simulink model "CompFilter_testHarness"  (R2012b)
settings: Solver=FixedStepDiscrete  StartTime=0.0  StopTime=50  RelTol=1e-3
InitFcn:
  | p = fileparts(which(bdroot));
  | load(fullfile(p,'CompFilter_testData'))
values from neighbouring files (symbols this model uses):
  F_LUT =     [CompFilter_testData.mat]    (also in filterResponseData.m = [])
undefined symbols (not defined in the file or in its folder): sigbuilder_block
libraries: simulink x13, ResultLoggerLib x4
settings Model: RequirementInfo={'other' '..\..\..\..\requirements\ebd_srs.doc' '@Simulink_requirement_item_4' 'true' 'REQ001- Filter input signal via polyphase digital filter bank' 'Requirement' } %GIDa_bfa4a348_cd9f_4101_a776_3ea215f34dae  SldvGeneratedHarnessModel=TestUnitModel=CompFeatures|  RecordCoverage=on  CovMetricSettings=dcmtroie  CovHTMLOptions=-sRT=1 -aTS=1 -bRG=1 -bTC=0 -hTR=0 -nFC=0 -scm=1 -bcm=1 -xEv=0  CovExternalEMLEnable=on  Creator=aanantha  LastModifiedBy=klindqvi
settings DataIOCC: SaveFormat=Structure  SignalLoggingSaveFormat=ModelDataLogs  SaveOutput=off  SaveTime=off  SignalLoggingName=logsOut
settings OptimizationCC: InlineParams=on  OptimizeModelRefInitCode=on  LifeSpan=1
settings DebuggingCC: ReadBeforeWriteMsg=DisableAll  WriteAfterWriteMsg=DisableAll  WriteAfterReadMsg=DisableAll  CheckSSInitialOutputMsg=off  SolverPrmCheckMsg=none  InheritedTsInSrcMsg=none  ParameterPrecisionLossMsg=none  FcnCallInpInsideContextMsg=EnableAllAsWarning  ModelReferenceSymbolNameMessage=none
settings HardwareCC: ProdLargestAtomicInteger=Long  ProdLargestAtomicFloat=Double  ProdEndianess=LittleEndian  ProdHWDeviceType=ARM Compatible->ARM Cortex
settings ModelReferenceCC: UpdateModelReferenceTargets=Force  CheckModelReferenceTargetMessage=none
settings RTWCC: SystemTargetFile=ert.tlc  TemplateMakefile=ert_default_tmf  Description=Embedded Coder  GenerateReport=on  ProcessScript=ert_make_rtw_hook  IncludeHyperlinkInReport=on  LaunchReport=on  GenerateTraceInfo=on  GenerateTraceReportSl=on  GenerateTraceReportSf=on  GenerateTraceReportEml=on  GenerateCodeMetricsReport=on
settings CodeAppCC: IgnoreCustomStorageClasses=off
settings ERTTargetCC: CodeReplacementLibrary=GCC ARM Cortex-A8  MultiwordLength=2048  GenerateSampleERTMain=on  ERTCustomFileTemplate=example_file_process.tlc  ConvertIfToSwitch=off  SuppressUnreachableDefaultCases=off

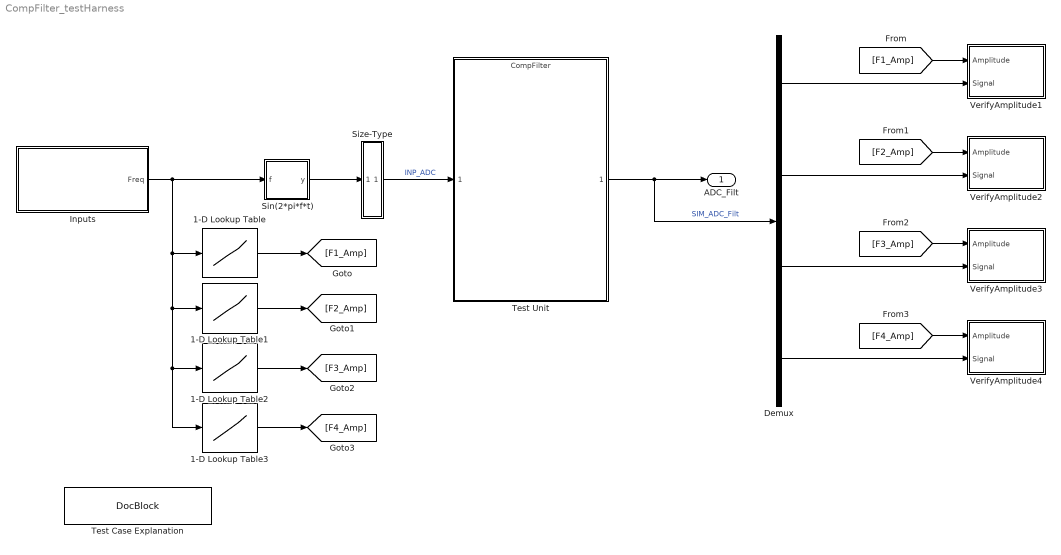
== system CompFilter_testHarness ==
  1-D Lookup Table : Lookup_n-D  NumberOfTableDimensions=1  BreakpointsForDimension1=F_LUT(1).bp  Table=F_LUT(1).table  InterpMethod=Cubic spline  RndMeth=Simplest  InputSameDT=on
  1-D Lookup Table1 : Lookup_n-D  NumberOfTableDimensions=1  BreakpointsForDimension1=F_LUT(2).bp  Table=F_LUT(2).table  InterpMethod=Cubic spline  RndMeth=Simplest  InputSameDT=on
  1-D Lookup Table2 : Lookup_n-D  NumberOfTableDimensions=1  BreakpointsForDimension1=F_LUT(3).bp  Table=F_LUT(3).table  InterpMethod=Cubic spline  RndMeth=Simplest  InputSameDT=on
  1-D Lookup Table3 : Lookup_n-D  NumberOfTableDimensions=1  BreakpointsForDimension1=F_LUT(4).bp  Table=F_LUT(4).table  InterpMethod=Cubic spline  RndMeth=Simplest  InputSameDT=on
  Demux : Demux
  Inputs : Subsystem  Tag=STV Subsys  RequirementInfo={'other' '..\..\..\..\requirements\ebd_srs.doc' '@REQ001- Filter input signal via polyphase digital filter bank' 'true' 'REQ001- Filter input signal via polyphase digital filter bank' '' ; 'other' '..\..\..\..\requirements\ebd_srs.doc' '@REQ001- Filter input signal via polyphase digital filter bank' 'true' 'REQ001- Filter input signal via polyphase digital filter bank' '' ; 'other' '..\..\..\..\requirements\ebd_srs.doc' '@REQ001- Filter input signal via polyphase digital filter bank' 'true' 'REQ001- Filter input signal via polyphase digital filter bank' '' ; 'other' '..\..\..\..\requirements\ebd_srs.doc' '@REQ001- Filter input signal via polyphase digital filter bank' 'true' 'REQ001- Filter input signal via polyphase digital filter bank' '' ; 'other' '..\..\..\..\requirements\ebd_srs.doc' '@REQ001- Filter input signal via polyphase digital filter bank' 'true' 'REQ001- Filter input signal via polyphase digital filter bank' '' ; 'other' '..\..\..\..\requirements\ebd_srs.doc' '@REQ001- Filter input signal via polyphase digital filter bank' 'true' 'REQ001- Filter input signal via polyphase digital filter bank' '' ; 'other' '..\..\..\..\requirements\ebd_srs.doc' '@REQ001- Filter input signal via polyphase digital filter bank' 'true' 'REQ001- Filter input signal via polyphase digital filter bank' '' } %GIDa_3ed100c0_3913_49f9_991c_94aec2cdfde7  LoadFcn=sigbuilder_block('load');  StartFcn=sigbuilder_block('start');  StopFcn=sigbuilder_block('stop');  ClipboardFcn=sigbuilder_block('clipboard');  mask(Sigbuilder block){}
      mask init:
      | if ~strcmp(get_param(bdroot(gcb),'SimulationStatus'),'stopped'),tuvar = sigbuilder_block('maskInit'); end
      settings: CopyFcn=sigbuilder_block('copy');  DeleteFcn=sigbuilder_block('delete');  ModelCloseFcn=sigbuilder_block('modelClose');  PreSaveFcn=sigbuilder_block('preSave');  PauseFcn=sigbuilder_block('pause');  ContinueFcn=sigbuilder_block('continue');  NameChangeFcn=sigbuilder_block('namechange');  OpenFcn=sigbuilder_block('open',[726.75 262.5 605.25 528 ]);  CloseFcn=sigbuilder_block('close');
      mask Display: plot(0, 0, 100, 100,[2, 2, 32, 32, 2], [68, 8, 8, 68, 68],[32, 2], [38, 38], [32, 19, 2],[53, 60, 44], [32, 17, 17, 2],[16, 16, 31, 31]);txt = getActiveGroup(gcbh);text(2, 100, txt,'verticalAlignment', 'top');
  Sin(2*pi*f*t) : Subsystem
  Size-Type : Subsystem
  Test Case Explanation : simulink/Model-Wide Utilities/DocBlock  DocumentType=Text
      content=|
      | Test case with default values because no SLDVDATA supplied
  Test Unit : ModelReference  ModelNameDialog=CompFilter  SimulationMode=Normal  ModelReferenceVersion=1.283  CopyOfModelName=CompFilter  DefaultDataLogging=on
  VerifyAmplitude1 : Subsystem
  VerifyAmplitude2 : Subsystem
  VerifyAmplitude3 : Subsystem
  VerifyAmplitude4 : Subsystem
  ADC_Filt : Outport  OutDataTypeStr=single  PortDimensions=4  SampleTime=[0.08900000000000001,0]
  wires:
  Size-Type/1(Out1) -> Test Unit/1  "INP_ADC"
  Test Unit/1 -> Demux/1, ADC_Filt/1  "SIM_ADC_Filt"
  [F1_Amp] -> VerifyAmplitude1/1(Amplitude)
  [F2_Amp] -> VerifyAmplitude2/1(Amplitude)
  Inputs/1(Freq) -> 1-D Lookup Table3/1, 1-D Lookup Table2/1, 1-D Lookup Table1/1, 1-D Lookup Table/1, Sin(2*pi*f*t)/1(f)
  Sin(2*pi*f*t)/1(y) -> Size-Type/1(In1)
  Demux/1 -> VerifyAmplitude1/2(Signal)
  Demux/2 -> VerifyAmplitude2/2(Signal)
  1-D Lookup Table/1 -> [F1_Amp]
  1-D Lookup Table1/1 -> [F2_Amp]
  1-D Lookup Table2/1 -> [F3_Amp]
  1-D Lookup Table3/1 -> [F4_Amp]
  Demux/3 -> VerifyAmplitude3/2(Signal)
  [F3_Amp] -> VerifyAmplitude3/1(Amplitude)
  [F4_Amp] -> VerifyAmplitude4/1(Amplitude)
  Demux/4 -> VerifyAmplitude4/2(Signal)

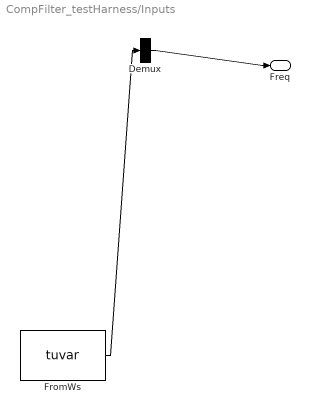
== system CompFilter_testHarness/Inputs ==
  Demux : Demux  Tag=STV Demux  Outputs=1
  FromWs : FromWorkspace  Tag=STV FromWs  VariableName=tuvar  SampleTime=0
      SigBuilderData=|
      | dataSet(1).timeRange = [0 50]
      | dataSet(1).name = 'Test Case 1'
      | dataSet(2).timeRange = [0 50]
      | dataSet(2).name = 'Test Case 2'
      | dataSet(3).timeRange = [0 50]
      | dataSet(3).name = 'Test Case 3'
      | dataSet(4).timeRange = [0 50]
      | dataSet(4).name = 'Test Case 4'
      | dataSet(5).timeRange = [0 50]
      | dataSet(5).name = 'Test Case 5'
      | dataSet(6).timeRange = [0 50]
      | dataSet(6).name = 'Test Case 6'
      | dataSet(7).timeRange = [0 50]
      | dataSet(7).name = 'Test Case 7'
      | sbobj.Name = 'Signal Builder'
      | sbobj.Groups(1).Name = 'Test Case 1'
      | sbobj.Groups(1).Signals.Name = 'Freq'
      | sbobj.Groups(1).Signals.XData = [0 50]
      | sbobj.Groups(1).Signals.YData = [10 10]
      | sbobj.Groups(1).TimeRange = [0 50]
      | sbobj.Groups(2).Name = 'Test Case 2'
      | sbobj.Groups(2).Signals.Name = 'Freq'
      | sbobj.Groups(2).Signals.XData = [0 50]
      | sbobj.Groups(2).Signals.YData = [1 1]
      | sbobj.Groups(2).TimeRange = [0 50]
      | sbobj.Groups(3).Name = 'Test Case 3'
      | sbobj.Groups(3).Signals.Name = 'Freq'
      | sbobj.Groups(3).Signals.XData = [0 50]
      | sbobj.Groups(3).Signals.YData = [5.6 5.6]
      | sbobj.Groups(3).TimeRange = [0 50]
      | sbobj.Groups(4).Name = 'Test Case 4'
      | sbobj.Groups(4).Signals.Name = 'Freq'
      | sbobj.Groups(4).Signals.XData = [0 50]
      | sbobj.Groups(4).Signals.YData = [10 10]
      | sbobj.Groups(4).TimeRange = [0 50]
      | sbobj.Groups(5).Name = 'Test Case 5'
      | sbobj.Groups(5).Signals.Name = 'Freq'
      | sbobj.Groups(5).Signals.XData = [0 50]
      | sbobj.Groups(5).Signals.YData = [15 15]
      | sbobj.Groups(5).TimeRange = [0 50]
      | sbobj.Groups(6).Name = 'Test Case 6'
      | sbobj.Groups(6).Signals.Name = 'Freq'
      | sbobj.Groups(6).Signals.XData = [0 50]
      | sbobj.Groups(6).Signals.YData = [20 20]
      | sbobj.Groups(6).TimeRange = [0 50]
      | sbobj.Groups(7).Name = 'Test Case 7'
      | sbobj.Groups(7).Signals.Name = 'Freq'
      | sbobj.Groups(7).Signals.XData = [0 50]
      | sbobj.Groups(7).Signals.YData = [100 100]
      | sbobj.Groups(7).TimeRange = [0 50]
  Freq : Outport  Tag=STV Outport
  wires:
  FromWs/1 -> Demux/1
  Demux/1 -> Freq/1

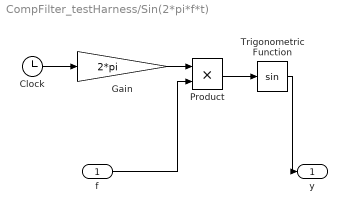
== system CompFilter_testHarness/Sin(2*pi*f*t) ==
  f : Inport
  Clock : Clock
  Gain : Gain  Gain=2*pi
  Product : Product  RndMeth=Zero
  Trigonometric Function : Trigonometry
  y : Outport
  wires:
  f/1 -> Product/2
  Clock/1 -> Gain/1
  Trigonometric Function/1 -> y/1
  Product/1 -> Trigonometric Function/1
  Gain/1 -> Product/1

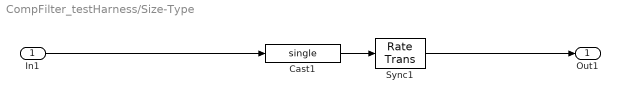
== system CompFilter_testHarness/Size-Type ==
  In1 : Inport
  Cast1 : DataTypeConversion  OutDataTypeStr=single  SaturateOnIntegerOverflow=on  RndMeth=Zero
  Sync1 : RateTransition  OutPortSampleTime=[0.001,0]
  Out1 : Outport
  wires:
  In1/1 -> Cast1/1
  Cast1/1 -> Sync1/1
  Sync1/1 -> Out1/1

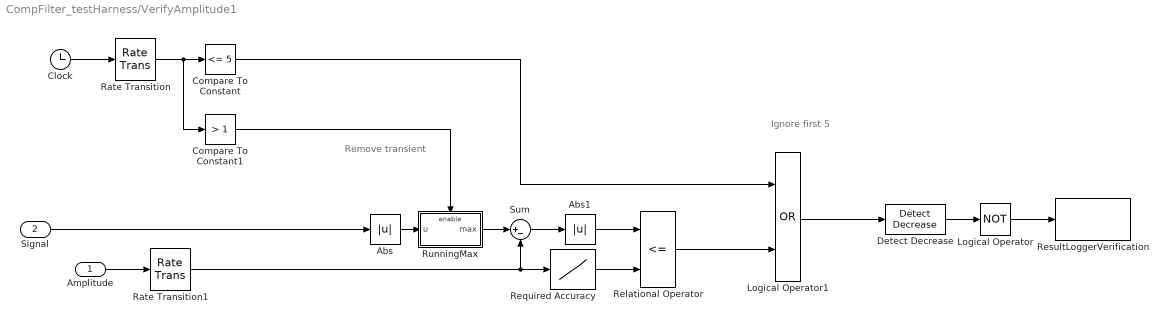
== system CompFilter_testHarness/VerifyAmplitude1 ==
  note: Remove transient
  note: Ignore first 5
  Amplitude : Inport
  Signal : Inport  Port=2
  Abs : Abs
  Abs1 : Abs
  Clock : Clock
  Compare To Constant : simulink/Logic and Bit Operations/Compare To Constant  relop=<=  const=5  OutDataTypeStr=boolean
  Compare To Constant1 : simulink/Logic and Bit Operations/Compare To Constant  relop=>  const=1  OutDataTypeStr=boolean
  Detect Decrease : simulink/Logic and Bit Operations/Detect Decrease  vinit=0.0  InputProcessing=Inherited  OutDataTypeStr=boolean
  Logical Operator : Logic  Operator=NOT  Inputs=1  AllPortsSameDT=off  OutDataTypeStr=boolean
  Logical Operator1 : Logic  Operator=OR  AllPortsSameDT=off  OutDataTypeStr=boolean
  Rate Transition : RateTransition  OutPortSampleTimeOpt=Inherit  OutPortSampleTime=0.089
  Rate Transition1 : RateTransition  OutPortSampleTime=0.089
  Relational Operator : RelationalOperator  Operator=<=  OutDataTypeStr=boolean
  Required Accuracy : Lookup_n-D  NumberOfTableDimensions=1  BreakpointsForDimension1=[0.05,2]  Table=[0.05,0.5]  ExtrapMethod=Clip  UseLastTableValue=on  RndMeth=Simplest  InputSameDT=on
  ResultLoggerVerification : ResultLoggerLib/ResultLoggerVerification  Description=Check for Feature 1 Amplitude Requirement  resultLoggerDescription=Check for Feature 1 Amplitude Requirement
      settings: AttributesFormatString=%<Description>
  RunningMax : Subsystem
  Sum : Sum  Inputs=|+-
  wires:
  Clock/1 -> Rate Transition/1
  Compare To Constant/1 -> Logical Operator1/1
  Detect Decrease/1 -> Logical Operator/1
  Logical Operator/1 -> ResultLoggerVerification/1
  Rate Transition/1 -> Compare To Constant1/1, Compare To Constant/1
  Signal/1 -> Abs/1
  Amplitude/1 -> Rate Transition1/1
  Logical Operator1/1 -> Detect Decrease/1
  Compare To Constant1/1 -> RunningMax/Enable
  Sum/1 -> Abs1/1
  Required Accuracy/1 -> Relational Operator/2
  Abs1/1 -> Relational Operator/1
  RunningMax/1(max) -> Sum/1
  Abs/1 -> RunningMax/1(u)
  Relational Operator/1 -> Logical Operator1/2
  Rate Transition1/1 -> Sum/2, Required Accuracy/1

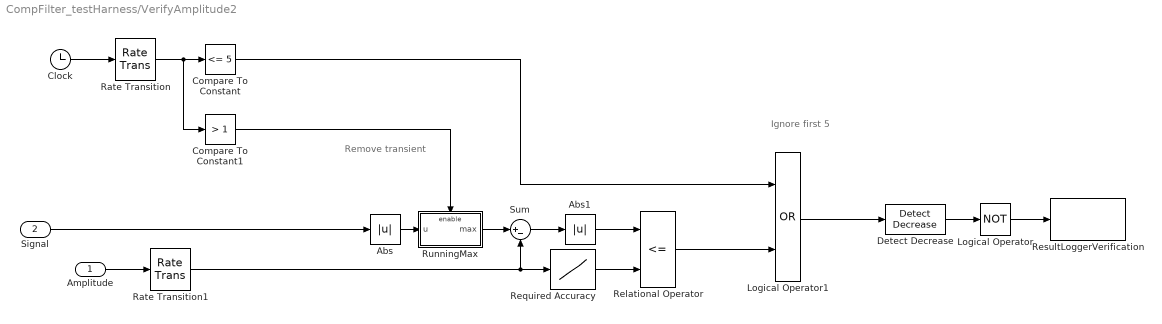
== system CompFilter_testHarness/VerifyAmplitude2 ==
  note: Ignore first 5
  note: Remove transient
  Amplitude : Inport
  Signal : Inport  Port=2
  Abs : Abs
  Abs1 : Abs
  Clock : Clock
  Compare To Constant : simulink/Logic and Bit Operations/Compare To Constant  relop=<=  const=5  OutDataTypeStr=boolean
  Compare To Constant1 : simulink/Logic and Bit Operations/Compare To Constant  relop=>  const=1  OutDataTypeStr=boolean
  Detect Decrease : simulink/Logic and Bit Operations/Detect Decrease  vinit=0.0  InputProcessing=Inherited  OutDataTypeStr=boolean
  Logical Operator : Logic  Operator=NOT  Inputs=1  AllPortsSameDT=off  OutDataTypeStr=boolean
  Logical Operator1 : Logic  Operator=OR  AllPortsSameDT=off  OutDataTypeStr=boolean
  Rate Transition : RateTransition  OutPortSampleTimeOpt=Inherit
  Rate Transition1 : RateTransition  OutPortSampleTimeOpt=Inherit
  Relational Operator : RelationalOperator  Operator=<=  OutDataTypeStr=boolean
  Required Accuracy : Lookup_n-D  NumberOfTableDimensions=1  BreakpointsForDimension1=[0.05,2]  Table=[0.05,0.5]  ExtrapMethod=Clip  UseLastTableValue=on  RndMeth=Simplest  InputSameDT=on
  ResultLoggerVerification : ResultLoggerLib/ResultLoggerVerification  Description=Check for Feature 2 Amplitude Requirement  resultLoggerDescription=Check for Feature 2 Amplitude Requirement
      settings: AttributesFormatString=%<Description>
  RunningMax : Subsystem
  Sum : Sum  Inputs=|+-
  wires:
  Relational Operator/1 -> Logical Operator1/2
  Abs/1 -> RunningMax/1(u)
  RunningMax/1(max) -> Sum/1
  Abs1/1 -> Relational Operator/1
  Required Accuracy/1 -> Relational Operator/2
  Sum/1 -> Abs1/1
  Compare To Constant1/1 -> RunningMax/Enable
  Logical Operator1/1 -> Detect Decrease/1
  Amplitude/1 -> Rate Transition1/1
  Signal/1 -> Abs/1
  Rate Transition/1 -> Compare To Constant/1, Compare To Constant1/1
  Logical Operator/1 -> ResultLoggerVerification/1
  Detect Decrease/1 -> Logical Operator/1
  Compare To Constant/1 -> Logical Operator1/1
  Clock/1 -> Rate Transition/1
  Rate Transition1/1 -> Required Accuracy/1, Sum/2

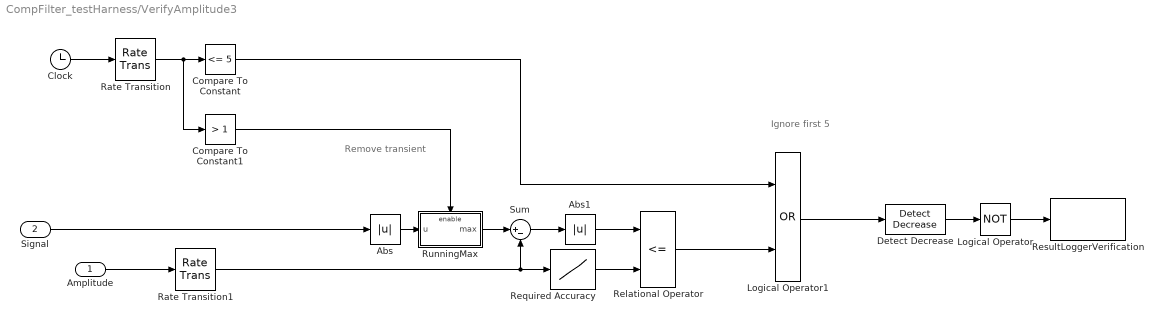
== system CompFilter_testHarness/VerifyAmplitude3 ==
  note: Remove transient
  note: Ignore first 5
  Amplitude : Inport
  Signal : Inport  Port=2
  Abs : Abs
  Abs1 : Abs
  Clock : Clock
  Compare To Constant : simulink/Logic and Bit Operations/Compare To Constant  relop=<=  const=5  OutDataTypeStr=boolean
  Compare To Constant1 : simulink/Logic and Bit Operations/Compare To Constant  relop=>  const=1  OutDataTypeStr=boolean
  Detect Decrease : simulink/Logic and Bit Operations/Detect Decrease  vinit=0.0  InputProcessing=Inherited  OutDataTypeStr=boolean
  Logical Operator : Logic  Operator=NOT  Inputs=1  AllPortsSameDT=off  OutDataTypeStr=boolean
  Logical Operator1 : Logic  Operator=OR  AllPortsSameDT=off  OutDataTypeStr=boolean
  Rate Transition : RateTransition  OutPortSampleTimeOpt=Inherit
  Rate Transition1 : RateTransition  OutPortSampleTimeOpt=Inherit
  Relational Operator : RelationalOperator  Operator=<=  OutDataTypeStr=boolean
  Required Accuracy : Lookup_n-D  NumberOfTableDimensions=1  BreakpointsForDimension1=[0.05,2]  Table=[0.05,0.5]  ExtrapMethod=Clip  UseLastTableValue=on  RndMeth=Simplest  InputSameDT=on
  ResultLoggerVerification : ResultLoggerLib/ResultLoggerVerification  Description=Check for Feature 3 Amplitude Requirement  resultLoggerDescription=Check for Feature 3 Amplitude Requirement
      settings: AttributesFormatString=%<Description>
  RunningMax : Subsystem
  Sum : Sum  Inputs=|+-
  wires:
  Clock/1 -> Rate Transition/1
  Compare To Constant/1 -> Logical Operator1/1
  Detect Decrease/1 -> Logical Operator/1
  Logical Operator/1 -> ResultLoggerVerification/1
  Rate Transition/1 -> Compare To Constant1/1, Compare To Constant/1
  Signal/1 -> Abs/1
  Amplitude/1 -> Rate Transition1/1
  Logical Operator1/1 -> Detect Decrease/1
  Compare To Constant1/1 -> RunningMax/Enable
  Sum/1 -> Abs1/1
  Required Accuracy/1 -> Relational Operator/2
  Abs1/1 -> Relational Operator/1
  RunningMax/1(max) -> Sum/1
  Abs/1 -> RunningMax/1(u)
  Relational Operator/1 -> Logical Operator1/2
  Rate Transition1/1 -> Sum/2, Required Accuracy/1

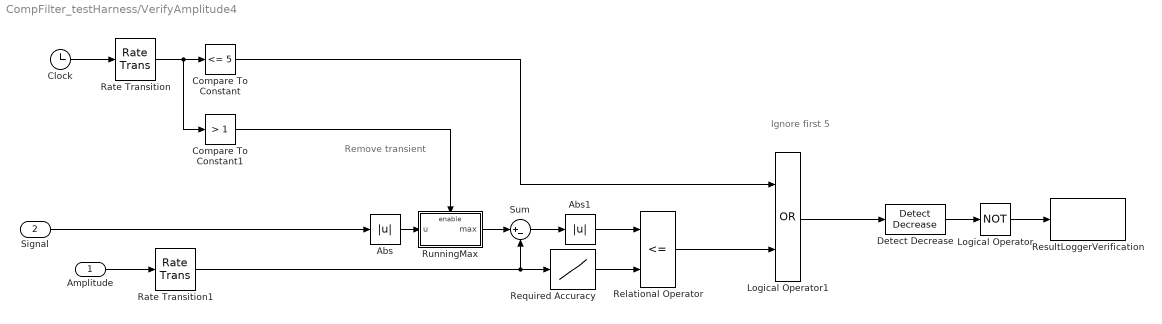
== system CompFilter_testHarness/VerifyAmplitude4 ==
  note: Ignore first 5
  note: Remove transient
  Amplitude : Inport
  Signal : Inport  Port=2
  Abs : Abs
  Abs1 : Abs
  Clock : Clock
  Compare To Constant : simulink/Logic and Bit Operations/Compare To Constant  relop=<=  const=5  OutDataTypeStr=boolean
  Compare To Constant1 : simulink/Logic and Bit Operations/Compare To Constant  relop=>  const=1  OutDataTypeStr=boolean
  Detect Decrease : simulink/Logic and Bit Operations/Detect Decrease  vinit=0.0  InputProcessing=Inherited  OutDataTypeStr=boolean
  Logical Operator : Logic  Operator=NOT  Inputs=1  AllPortsSameDT=off  OutDataTypeStr=boolean
  Logical Operator1 : Logic  Operator=OR  AllPortsSameDT=off  OutDataTypeStr=boolean
  Rate Transition : RateTransition  OutPortSampleTimeOpt=Inherit
  Rate Transition1 : RateTransition  OutPortSampleTimeOpt=Inherit
  Relational Operator : RelationalOperator  Operator=<=  OutDataTypeStr=boolean
  Required Accuracy : Lookup_n-D  NumberOfTableDimensions=1  BreakpointsForDimension1=[0.05,2]  Table=[0.05,0.5]  ExtrapMethod=Clip  UseLastTableValue=on  RndMeth=Simplest  InputSameDT=on
  ResultLoggerVerification : ResultLoggerLib/ResultLoggerVerification  Description=Check for Feature 4 Amplitude Requirement  resultLoggerDescription=Check for Feature 4 Amplitude Requirement
      settings: AttributesFormatString=%<Description>
  RunningMax : Subsystem
  Sum : Sum  Inputs=|+-
  wires:
  Relational Operator/1 -> Logical Operator1/2
  Abs/1 -> RunningMax/1(u)
  RunningMax/1(max) -> Sum/1
  Abs1/1 -> Relational Operator/1
  Required Accuracy/1 -> Relational Operator/2
  Sum/1 -> Abs1/1
  Compare To Constant1/1 -> RunningMax/Enable
  Logical Operator1/1 -> Detect Decrease/1
  Amplitude/1 -> Rate Transition1/1
  Signal/1 -> Abs/1
  Rate Transition/1 -> Compare To Constant/1, Compare To Constant1/1
  Logical Operator/1 -> ResultLoggerVerification/1
  Detect Decrease/1 -> Logical Operator/1
  Compare To Constant/1 -> Logical Operator1/1
  Clock/1 -> Rate Transition/1
  Rate Transition1/1 -> Required Accuracy/1, Sum/2

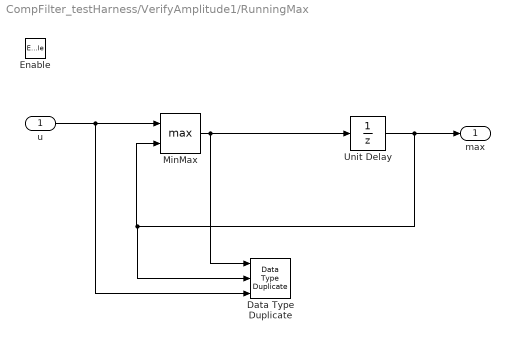
== system CompFilter_testHarness/VerifyAmplitude1/RunningMax ==
  u : Inport
  Enable : EnablePort
  Data Type Duplicate : DataTypeDuplicate  DisableCoverage=on  NumInputPorts=3
  MinMax : MinMax  DisableCoverage=on  Function=max  Inputs=2  OutDataTypeStr=Inherit: Inherit via back propagation  ZeroCross=off
      settings: LockScale=on
  Unit Delay : UnitDelay  SampleTime=-1
  max : Outport
  wires:
  u/1 -> MinMax/1, Data Type Duplicate/3
  MinMax/1 -> Unit Delay/1, Data Type Duplicate/1
  Unit Delay/1 -> Data Type Duplicate/2, MinMax/2, max/1

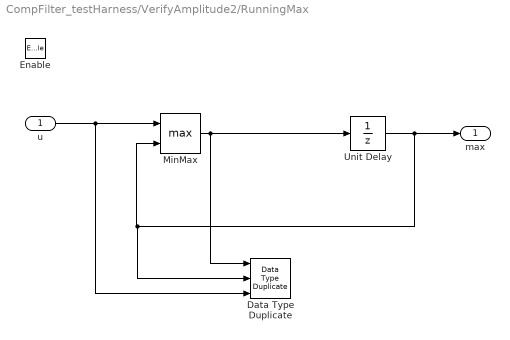
== system CompFilter_testHarness/VerifyAmplitude2/RunningMax ==
  u : Inport
  Enable : EnablePort
  Data Type Duplicate : DataTypeDuplicate  DisableCoverage=on  NumInputPorts=3
  MinMax : MinMax  DisableCoverage=on  Function=max  Inputs=2  OutDataTypeStr=Inherit: Inherit via back propagation  ZeroCross=off
      settings: LockScale=on
  Unit Delay : UnitDelay  SampleTime=-1
  max : Outport
  wires:
  Unit Delay/1 -> max/1, MinMax/2, Data Type Duplicate/2
  MinMax/1 -> Data Type Duplicate/1, Unit Delay/1
  u/1 -> Data Type Duplicate/3, MinMax/1

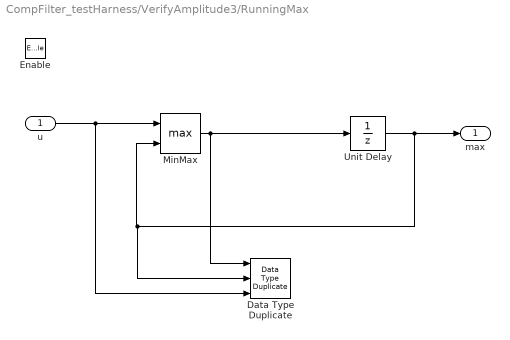
== system CompFilter_testHarness/VerifyAmplitude3/RunningMax ==
  u : Inport
  Enable : EnablePort
  Data Type Duplicate : DataTypeDuplicate  DisableCoverage=on  NumInputPorts=3
  MinMax : MinMax  DisableCoverage=on  Function=max  Inputs=2  OutDataTypeStr=Inherit: Inherit via back propagation  ZeroCross=off
      settings: LockScale=on
  Unit Delay : UnitDelay  SampleTime=-1
  max : Outport
  wires:
  u/1 -> MinMax/1, Data Type Duplicate/3
  MinMax/1 -> Unit Delay/1, Data Type Duplicate/1
  Unit Delay/1 -> Data Type Duplicate/2, MinMax/2, max/1

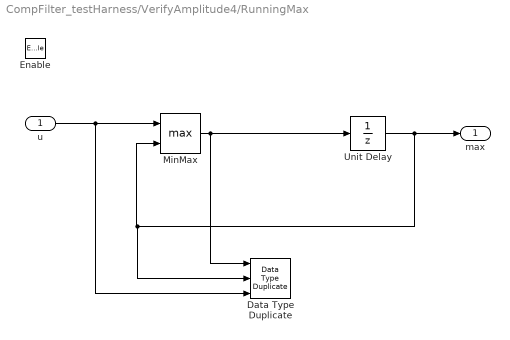
== system CompFilter_testHarness/VerifyAmplitude4/RunningMax ==
  u : Inport
  Enable : EnablePort
  Data Type Duplicate : DataTypeDuplicate  DisableCoverage=on  NumInputPorts=3
  MinMax : MinMax  DisableCoverage=on  Function=max  Inputs=2  OutDataTypeStr=Inherit: Inherit via back propagation  ZeroCross=off
      settings: LockScale=on
  Unit Delay : UnitDelay  SampleTime=-1
  max : Outport
  wires:
  Unit Delay/1 -> max/1, MinMax/2, Data Type Duplicate/2
  MinMax/1 -> Data Type Duplicate/1, Unit Delay/1
  u/1 -> Data Type Duplicate/3, MinMax/1
